simulink model "my_model"  (R2020b)
settings: Solver=VariableStepAuto  StartTime=0.0  StopTime=10.0  RelTol=1e-3
settings Model: Creator=morro  LastModifiedBy=morro

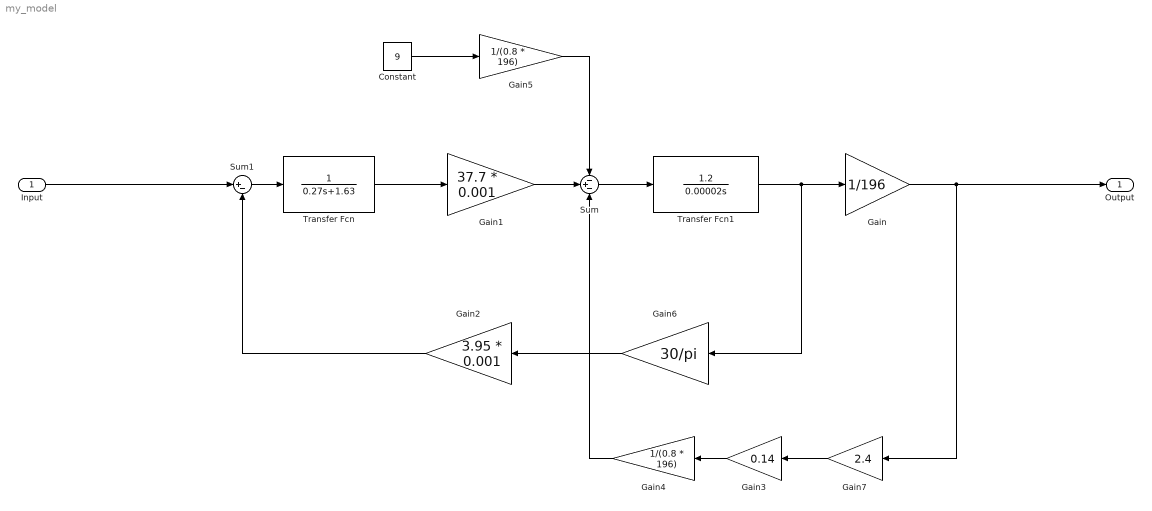
== system my_model ==
  Input : Inport
  Constant : Constant  Value=9
  Gain : Gain  Gain=1/196
  Gain1 : Gain  Gain=37.7 * 0.001
  Gain2 : Gain  Gain=3.95 * 0.001
  Gain3 : Gain  Gain=0.14
  Gain4 : Gain  Gain=1/(0.8 * 196)
  Gain5 : Gain  Gain=1/(0.8 * 196)
  Gain6 : Gain  Gain=30/pi
  Gain7 : Gain  Gain=2.4
  Sum : Sum  Inputs=-+-
  Sum1 : Sum  Inputs=|+-
  Transfer Fcn : TransferFcn  Denominator=[0.27 1.63]
  Transfer Fcn1 : TransferFcn  Numerator=[1.2]  Denominator=[0.00002 0]
  Output : Outport
  wires:
  Input/1 -> Sum1/1
  Gain6/1 -> Gain2/1
  Constant/1 -> Gain5/1
  Sum/1 -> Transfer Fcn1/1
  Gain1/1 -> Sum/2
  Gain4/1 -> Sum/3
  Gain2/1 -> Sum1/2
  Gain7/1 -> Gain3/1
  Sum1/1 -> Transfer Fcn/1
  Transfer Fcn/1 -> Gain1/1
  Gain3/1 -> Gain4/1
  Transfer Fcn1/1 -> Gain6/1, Gain/1
  Gain5/1 -> Sum/1
  Gain/1 -> Output/1, Gain7/1
